simulink model "iris_layer1_rvco_16"  (R2023b)
settings: Solver=VariableStepAuto  StartTime=0.0  StopTime=10.0  RelTol=1e-3
libraries: vco_snn x16, dspswit3 x16, spspowerguiLib x1
settings Model: Creator=saisanjeet  LastModifiedBy=saisanjeet

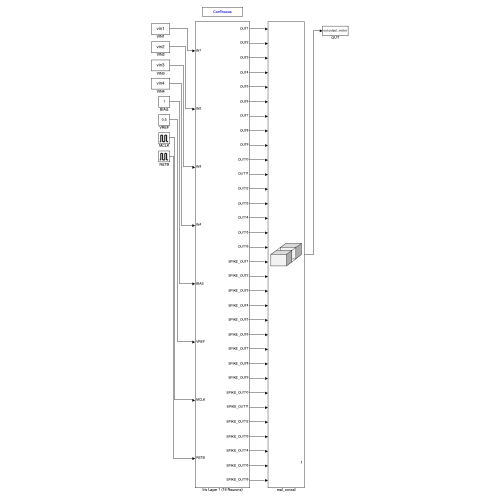
[thumbnail: Simulink's stored preview of the top-level diagram]
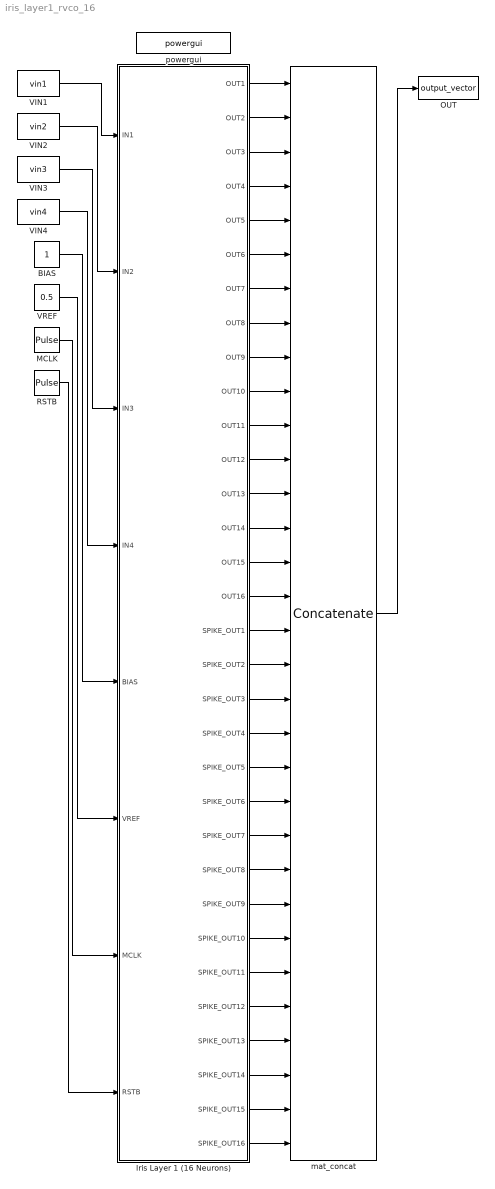
== system iris_layer1_rvco_16 ==
  BIAS : Constant
  Iris Layer 1 (16 Neurons) : Subsystem
  MCLK : DiscretePulseGenerator  PulseType=Time based  Period=1e-08  PulseWidth=50  PhaseDelay=1e-09
  OUT : ToWorkspace  VariableName=output_vector  SaveFormat=Timeseries  SampleTime=-1
  RSTB : DiscretePulseGenerator  PulseType=Time based  Period=4.02e-06  PulseWidth=99  PhaseDelay=1e-09
  VIN1 : FromWorkspace  VariableName=vin1  Interpolate=off  OutputAfterFinalValue=Setting to zero
  VIN2 : FromWorkspace  VariableName=vin2  Interpolate=off  OutputAfterFinalValue=Setting to zero
  VIN3 : FromWorkspace  VariableName=vin3  Interpolate=off  OutputAfterFinalValue=Setting to zero
  VIN4 : FromWorkspace  VariableName=vin4  Interpolate=off  OutputAfterFinalValue=Setting to zero
  VREF : Constant  Value=0.5
  mat_concat : Concatenate  NumInputs=32  Mode=Multidimensional array
  powergui : spspowerguiLib/powergui  Priority=1  SimulationMode=Continuous  SampleTime=50e-6  frequency=60  Iterations=50  frequencyindice=60  Pbase=100e6  ErrMax=1e-4  UnitsV=kV  UnitsW=MW  buscounter=0  FunctionMessages=off  echomessages=off  EnableUseOfTLC=off  CurrentSourceSwitches=off  DisableSnubberDevices=off  DisableRonSwitches=off  DisableVfSwitches=off  DisplayEquations=off  AutomaticDiscreteSolvers=off  SolverType=Tustin/Backward Euler (TBE)  Interpol=off  ExternalGateDelay=off  methode=off  Ts=100  x0status=blocks  SPID=on  SwTol=0  HookPort=off  NonlinearTolerance=1e-4  nMaxIteration=100  ContinueOnMaxIteration=off  RestoreLinks=warning  ResistiveCurrentMeasurement=off  Frange=[0:2:500]  Ylog=off  Xlog=on  ShowGrid=off  save=off  variable=ZData  structure=0  ZoomFFT=off  StartTime=0.0  cycles=1  DisplayStyle=1  fundamental=60  FreqAxis=off  MaxFrequency=1000  frequencyindicesteady=1  RmsSteady=1  display=off
  wires:
  VIN1/1 -> Iris Layer 1 (16 Neurons)/1(IN1)
  VIN2/1 -> Iris Layer 1 (16 Neurons)/2(IN2)
  VIN3/1 -> Iris Layer 1 (16 Neurons)/3(IN3)
  VIN4/1 -> Iris Layer 1 (16 Neurons)/4(IN4)
  BIAS/1 -> Iris Layer 1 (16 Neurons)/5(BIAS)
  VREF/1 -> Iris Layer 1 (16 Neurons)/6(VREF)
  MCLK/1 -> Iris Layer 1 (16 Neurons)/7(MCLK)
  RSTB/1 -> Iris Layer 1 (16 Neurons)/8(RSTB)
  Iris Layer 1 (16 Neurons)/1(OUT1) -> mat_concat/1
  Iris Layer 1 (16 Neurons)/17(SPIKE_OUT1) -> mat_concat/17
  Iris Layer 1 (16 Neurons)/2(OUT2) -> mat_concat/2
  Iris Layer 1 (16 Neurons)/18(SPIKE_OUT2) -> mat_concat/18
  Iris Layer 1 (16 Neurons)/3(OUT3) -> mat_concat/3
  Iris Layer 1 (16 Neurons)/19(SPIKE_OUT3) -> mat_concat/19
  Iris Layer 1 (16 Neurons)/4(OUT4) -> mat_concat/4
  Iris Layer 1 (16 Neurons)/20(SPIKE_OUT4) -> mat_concat/20
  Iris Layer 1 (16 Neurons)/5(OUT5) -> mat_concat/5
  Iris Layer 1 (16 Neurons)/21(SPIKE_OUT5) -> mat_concat/21
  Iris Layer 1 (16 Neurons)/6(OUT6) -> mat_concat/6
  Iris Layer 1 (16 Neurons)/22(SPIKE_OUT6) -> mat_concat/22
  Iris Layer 1 (16 Neurons)/7(OUT7) -> mat_concat/7
  Iris Layer 1 (16 Neurons)/23(SPIKE_OUT7) -> mat_concat/23
  Iris Layer 1 (16 Neurons)/8(OUT8) -> mat_concat/8
  Iris Layer 1 (16 Neurons)/24(SPIKE_OUT8) -> mat_concat/24
  Iris Layer 1 (16 Neurons)/9(OUT9) -> mat_concat/9
  Iris Layer 1 (16 Neurons)/25(SPIKE_OUT9) -> mat_concat/25
  Iris Layer 1 (16 Neurons)/10(OUT10) -> mat_concat/10
  Iris Layer 1 (16 Neurons)/26(SPIKE_OUT10) -> mat_concat/26
  Iris Layer 1 (16 Neurons)/11(OUT11) -> mat_concat/11
  Iris Layer 1 (16 Neurons)/27(SPIKE_OUT11) -> mat_concat/27
  Iris Layer 1 (16 Neurons)/12(OUT12) -> mat_concat/12
  Iris Layer 1 (16 Neurons)/28(SPIKE_OUT12) -> mat_concat/28
  Iris Layer 1 (16 Neurons)/13(OUT13) -> mat_concat/13
  Iris Layer 1 (16 Neurons)/29(SPIKE_OUT13) -> mat_concat/29
  Iris Layer 1 (16 Neurons)/14(OUT14) -> mat_concat/14
  Iris Layer 1 (16 Neurons)/30(SPIKE_OUT14) -> mat_concat/30
  Iris Layer 1 (16 Neurons)/15(OUT15) -> mat_concat/15
  Iris Layer 1 (16 Neurons)/31(SPIKE_OUT15) -> mat_concat/31
  Iris Layer 1 (16 Neurons)/16(OUT16) -> mat_concat/16
  Iris Layer 1 (16 Neurons)/32(SPIKE_OUT16) -> mat_concat/32
  mat_concat/1 -> OUT/1

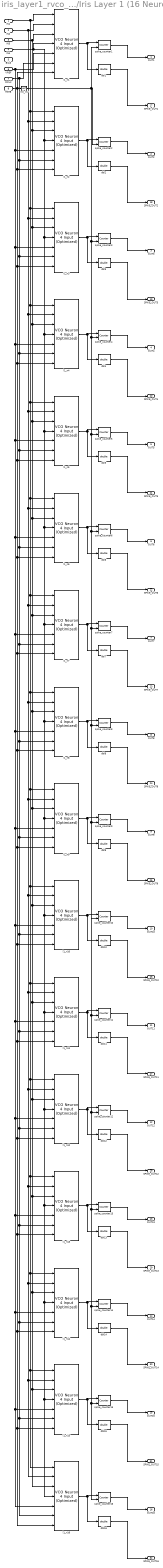
== system iris_layer1_rvco_16/Iris Layer 1 (16 Neurons) ==
  IN1 : Inport
  IN2 : Inport  Port=2
  IN3 : Inport  Port=3
  IN4 : Inport  Port=4
  BIAS : Inport  Port=5
  VREF : Inport  Port=6
  MCLK : Inport  Port=7
  RSTB : Inport  Port=8
  dbl{1..16} (16 alike) : DataTypeConversion  OutDataTypeStr=double  SaturateOnIntegerOverflow=off  RndMeth=Floor
  l1_n1 : vco_snn/VCO Neuron 4 Input (Optimized)  kvco=10000000  center_freq=100000000  xor_tau=1.5e-09  rf=50000  vth=0.4  vcm=0.5  spike_amp=0.2  rin1=19778.2852  spike_sign1=1  rin2=21811.0078  spike_sign2=-1  rin3=46837.6719  spike_sign3=-1  rin4=22517.3164  spike_sign4=1
  l1_n10 : vco_snn/VCO Neuron 4 Input (Optimized)  kvco=10000000  center_freq=100000000  xor_tau=1.5e-09  rf=50000  vth=0.4  vcm=0.5  spike_amp=0.2  rin1=11850.6855  spike_sign1=1  rin2=94836.5  spike_sign2=-1  rin3=21873.4844  spike_sign3=1  rin4=23860.0938  spike_sign4=-1
  l1_n11 : vco_snn/VCO Neuron 4 Input (Optimized)  kvco=10000000  center_freq=100000000  xor_tau=1.5e-09  rf=50000  vth=0.4  vcm=0.5  spike_amp=0.2  rin1=11218.9355  spike_sign1=1  rin2=22596.9961  spike_sign2=-1  rin3=15442.873  spike_sign3=1  rin4=740390.1875  spike_sign4=-1
  l1_n12 : vco_snn/VCO Neuron 4 Input (Optimized)  kvco=10000000  center_freq=100000000  xor_tau=1.5e-09  rf=50000  vth=0.4  vcm=0.5  spike_amp=0.2  rin1=19495.0039  spike_sign1=-1  rin2=17672.1855  spike_sign2=1  rin3=18269.4512  spike_sign3=-1  rin4=50958.6992  spike_sign4=1
  l1_n13 : vco_snn/VCO Neuron 4 Input (Optimized)  kvco=10000000  center_freq=100000000  xor_tau=1.5e-09  rf=50000  vth=0.4  vcm=0.5  spike_amp=0.2  rin1=35862.4062  spike_sign1=-1  rin2=97024.5547  spike_sign2=-1  rin3=10815.8164  spike_sign3=-1  rin4=23630.8555  spike_sign4=-1
  l1_n14 : vco_snn/VCO Neuron 4 Input (Optimized)  kvco=10000000  center_freq=100000000  xor_tau=1.5e-09  rf=50000  vth=0.4  vcm=0.5  spike_amp=0.2  rin1=19686.9551  spike_sign1=1  rin2=59508.957  spike_sign2=-1  rin3=12421.2666  spike_sign3=1  rin4=18954.0312  spike_sign4=1
  l1_n15 : vco_snn/VCO Neuron 4 Input (Optimized)  kvco=10000000  center_freq=100000000  xor_tau=1.5e-09  rf=50000  vth=0.4  vcm=0.5  spike_amp=0.2  rin1=137965.4844  spike_sign1=-1  rin2=14123.9453  spike_sign2=-1  rin3=17121.0996  spike_sign3=1  rin4=31897.6289  spike_sign4=1
  l1_n16 : vco_snn/VCO Neuron 4 Input (Optimized)  kvco=10000000  center_freq=100000000  xor_tau=1.5e-09  rf=50000  vth=0.4  vcm=0.5  spike_amp=0.2  rin1=16056.2139  spike_sign1=-1  rin2=15486.3701  spike_sign2=1  rin3=17269.7656  spike_sign3=1  rin4=13269.0547  spike_sign4=1
  l1_n2 : vco_snn/VCO Neuron 4 Input (Optimized)  kvco=10000000  center_freq=100000000  xor_tau=1.5e-09  rf=50000  vth=0.4  vcm=0.5  spike_amp=0.2  rin1=10688.1436  spike_sign1=-1  rin2=16196.8242  spike_sign2=1  rin3=43679.5938  spike_sign3=-1  rin4=24670.3125  spike_sign4=1
  l1_n3 : vco_snn/VCO Neuron 4 Input (Optimized)  kvco=10000000  center_freq=100000000  xor_tau=1.5e-09  rf=50000  vth=0.4  vcm=0.5  spike_amp=0.2  rin1=63517.8945  spike_sign1=1  rin2=125955.5859  spike_sign2=-1  rin3=36891.3555  spike_sign3=1  rin4=143862.1875  spike_sign4=1
  l1_n4 : vco_snn/VCO Neuron 4 Input (Optimized)  kvco=10000000  center_freq=100000000  xor_tau=1.5e-09  rf=50000  vth=0.4  vcm=0.5  spike_amp=0.2  rin1=26604.0039  spike_sign1=1  rin2=29810.457  spike_sign2=-1  rin3=139403.2656  spike_sign3=-1  rin4=80537.0391  spike_sign4=-1
  l1_n5 : vco_snn/VCO Neuron 4 Input (Optimized)  kvco=10000000  center_freq=100000000  xor_tau=1.5e-09  rf=50000  vth=0.4  vcm=0.5  spike_amp=0.2  rin1=105372.3438  spike_sign1=1  rin2=134152.1406  spike_sign2=-1  rin3=12321.7383  spike_sign3=1  rin4=32313.4883  spike_sign4=1
  l1_n6 : vco_snn/VCO Neuron 4 Input (Optimized)  kvco=10000000  center_freq=100000000  xor_tau=1.5e-09  rf=50000  vth=0.4  vcm=0.5  spike_amp=0.2  rin1=27070.5605  spike_sign1=-1  rin2=16986.3926  spike_sign2=-1  rin3=61271.7969  spike_sign3=-1  rin4=25541.8984  spike_sign4=-1
  l1_n7 : vco_snn/VCO Neuron 4 Input (Optimized)  kvco=10000000  center_freq=100000000  xor_tau=1.5e-09  rf=50000  vth=0.4  vcm=0.5  spike_amp=0.2  rin1=32799.8711  spike_sign1=-1  rin2=131961.5156  spike_sign2=1  rin3=17100.5859  spike_sign3=1  rin4=20953.6133  spike_sign4=1
  l1_n8 : vco_snn/VCO Neuron 4 Input (Optimized)  kvco=10000000  center_freq=100000000  xor_tau=1.5e-09  rf=50000  vth=0.4  vcm=0.5  spike_amp=0.2  rin1=9945.3809  spike_sign1=-1  rin2=17866.4766  spike_sign2=1  rin3=37977.7383  spike_sign3=1  rin4=11168.9385  spike_sign4=1
  l1_n9 : vco_snn/VCO Neuron 4 Input (Optimized)  kvco=10000000  center_freq=100000000  xor_tau=1.5e-09  rf=50000  vth=0.4  vcm=0.5  spike_amp=0.2  rin1=15401.373  spike_sign1=1  rin2=11706.7979  spike_sign2=-1  rin3=10476.6729  spike_sign3=-1  rin4=19190.5449  spike_sign4=-1
  rst_inv : Logic  Operator=NOT  IconShape=distinctive  AllPortsSameDT=off  OutDataTypeStr=boolean
  spike_counter{1..16} (16 alike) : dspswit3/Counter  Direction=Up  CountEvent=Rising edge  CounterSize=User defined  MaxCount=1024  InitialCount=0  Output=Count  HitValue=32  ResetInput=on  SamplesPerFrame=1  Ts=1  CntDtype=double  HitDtype=Logical
  OUT1 : Outport
  OUT2 : Outport  Port=2
  OUT3 : Outport  Port=3
  OUT4 : Outport  Port=4
  OUT5 : Outport  Port=5
  OUT6 : Outport  Port=6
  OUT7 : Outport  Port=7
  OUT8 : Outport  Port=8
  OUT9 : Outport  Port=9
  OUT10 : Outport  Port=10
  OUT11 : Outport  Port=11
  OUT12 : Outport  Port=12
  OUT13 : Outport  Port=13
  OUT14 : Outport  Port=14
  OUT15 : Outport  Port=15
  OUT16 : Outport  Port=16
  SPIKE_OUT1 : Outport  Port=17
  SPIKE_OUT2 : Outport  Port=18
  SPIKE_OUT3 : Outport  Port=19
  SPIKE_OUT4 : Outport  Port=20
  SPIKE_OUT5 : Outport  Port=21
  SPIKE_OUT6 : Outport  Port=22
  SPIKE_OUT7 : Outport  Port=23
  SPIKE_OUT8 : Outport  Port=24
  SPIKE_OUT9 : Outport  Port=25
  SPIKE_OUT10 : Outport  Port=26
  SPIKE_OUT11 : Outport  Port=27
  SPIKE_OUT12 : Outport  Port=28
  SPIKE_OUT13 : Outport  Port=29
  SPIKE_OUT14 : Outport  Port=30
  SPIKE_OUT15 : Outport  Port=31
  SPIKE_OUT16 : Outport  Port=32
  wires:
  dbl9/1 -> SPIKE_OUT9/1
  dbl5/1 -> SPIKE_OUT5/1
  dbl3/1 -> SPIKE_OUT3/1
  dbl11/1 -> SPIKE_OUT11/1
  spike_counter7/1 -> OUT7/1
  dbl12/1 -> SPIKE_OUT12/1
  dbl1/1 -> SPIKE_OUT1/1
  spike_counter13/1 -> OUT13/1
  spike_counter11/1 -> OUT11/1
  dbl15/1 -> SPIKE_OUT15/1
  spike_counter10/1 -> OUT10/1
  spike_counter8/1 -> OUT8/1
  dbl7/1 -> SPIKE_OUT7/1
  l1_n2/1 -> spike_counter2/1, dbl2/1
  l1_n13/1 -> spike_counter13/1, dbl13/1
  spike_counter12/1 -> OUT12/1
  spike_counter6/1 -> OUT6/1
  spike_counter2/1 -> OUT2/1
  spike_counter9/1 -> OUT9/1
  spike_counter3/1 -> OUT3/1
  l1_n4/1 -> spike_counter4/1, dbl4/1
  l1_n5/1 -> spike_counter5/1, dbl5/1
  dbl14/1 -> SPIKE_OUT14/1
  l1_n10/1 -> spike_counter10/1, dbl10/1
  dbl16/1 -> SPIKE_OUT16/1
  dbl6/1 -> SPIKE_OUT6/1
  l1_n1/1 -> spike_counter1/1, dbl1/1
  IN3/1 -> l1_n15/3, l1_n16/3, l1_n14/3, l1_n13/3, l1_n12/3, l1_n11/3, l1_n10/3, l1_n9/3, l1_n8/3, l1_n7/3, l1_n6/3, l1_n5/3, l1_n4/3, l1_n3/3, l1_n2/3, l1_n1/3
  l1_n6/1 -> spike_counter6/1, dbl6/1
  l1_n11/1 -> spike_counter11/1, dbl11/1
  l1_n14/1 -> spike_counter14/1, dbl14/1
  l1_n8/1 -> spike_counter8/1, dbl8/1
  l1_n12/1 -> spike_counter12/1, dbl12/1
  l1_n16/1 -> spike_counter16/1, dbl16/1
  spike_counter4/1 -> OUT4/1
  rst_inv/1 -> spike_counter15/2, spike_counter16/2, spike_counter14/2, spike_counter13/2, spike_counter12/2, spike_counter11/2, spike_counter9/2, spike_counter10/2, spike_counter8/2, spike_counter7/2, spike_counter6/2, spike_counter5/2, spike_counter4/2, spike_counter3/2, spike_counter1/2, spike_counter2/2
  spike_counter14/1 -> OUT14/1
  dbl13/1 -> SPIKE_OUT13/1
  VREF/1 -> l1_n15/5, l1_n16/5, l1_n14/5, l1_n13/5, l1_n12/5, l1_n11/5, l1_n10/5, l1_n9/5, l1_n8/5, l1_n7/5, l1_n6/5, l1_n5/5, l1_n4/5, l1_n3/5, l1_n2/5, l1_n1/5
  l1_n15/1 -> spike_counter15/1, dbl15/1
  RSTB/1 -> l1_n15/7, l1_n16/7, l1_n14/7, l1_n13/7, l1_n12/7, l1_n11/7, l1_n10/7, l1_n9/7, l1_n8/7, l1_n7/7, l1_n6/7, l1_n5/7, l1_n4/7, l1_n3/7, l1_n2/7, rst_inv/1, l1_n1/7
  dbl2/1 -> SPIKE_OUT2/1
  spike_counter15/1 -> OUT15/1
  spike_counter1/1 -> OUT1/1
  IN1/1 -> l1_n15/1, l1_n16/1, l1_n14/1, l1_n13/1, l1_n12/1, l1_n11/1, l1_n10/1, l1_n9/1, l1_n8/1, l1_n7/1, l1_n6/1, l1_n5/1, l1_n4/1, l1_n3/1, l1_n2/1, l1_n1/1
  IN2/1 -> l1_n15/2, l1_n16/2, l1_n14/2, l1_n13/2, l1_n12/2, l1_n11/2, l1_n10/2, l1_n9/2, l1_n8/2, l1_n7/2, l1_n6/2, l1_n5/2, l1_n4/2, l1_n3/2, l1_n2/2, l1_n1/2
  l1_n7/1 -> spike_counter7/1, dbl7/1
  spike_counter16/1 -> OUT16/1
  MCLK/1 -> l1_n15/6, l1_n16/6, l1_n14/6, l1_n13/6, l1_n12/6, l1_n11/6, l1_n10/6, l1_n9/6, l1_n8/6, l1_n7/6, l1_n6/6, l1_n5/6, l1_n4/6, l1_n3/6, l1_n2/6, l1_n1/6
  dbl4/1 -> SPIKE_OUT4/1
  IN4/1 -> l1_n15/4, l1_n16/4, l1_n14/4, l1_n13/4, l1_n12/4, l1_n11/4, l1_n10/4, l1_n9/4, l1_n8/4, l1_n7/4, l1_n6/4, l1_n5/4, l1_n4/4, l1_n3/4, l1_n2/4, l1_n1/4
  l1_n3/1 -> spike_counter3/1, dbl3/1
  l1_n9/1 -> spike_counter9/1, dbl9/1
  dbl10/1 -> SPIKE_OUT10/1
  dbl8/1 -> SPIKE_OUT8/1
  spike_counter5/1 -> OUT5/1
